simulink model "bat_cap_discharge"  (R2023a)
settings: Solver=VariableStepAuto  StartTime=0.0  StopTime=110  RelTol=1e-3
undefined symbols (not defined in the file or in its folder): Battery, Capacitor, Ri
libraries: fl_lib x41, nesl_utility x22, batteryecm_lib x1
settings Model: Creator=antaeug  LastModifiedBy=antaeug

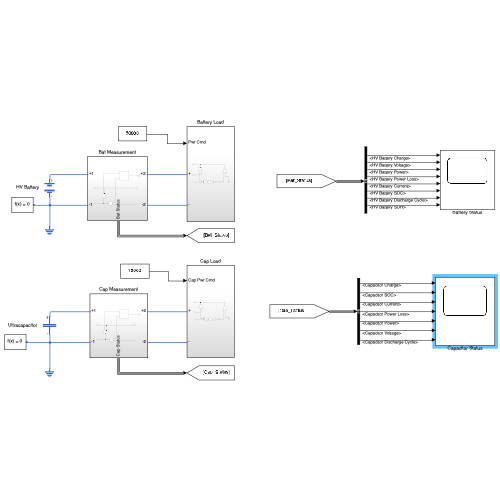
[thumbnail: Simulink's stored preview of the top-level diagram]
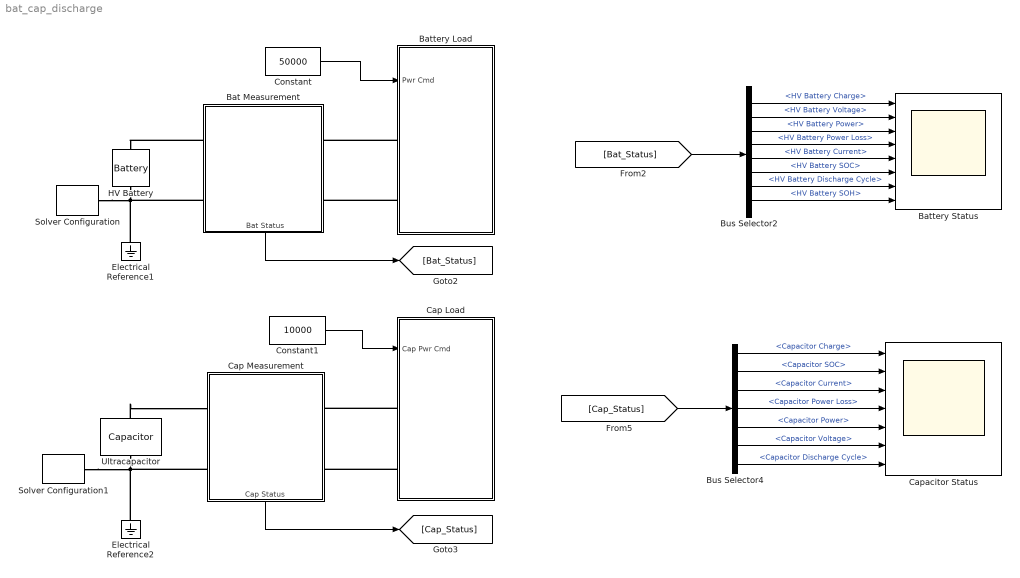
== system bat_cap_discharge ==
  Bat Measurement : Subsystem
      settings: PortSchema="{\"entries\":[{\"content\":{\"sides\":[{\"content\":{\"connectorIds\":[\"LConn1\",\"LConn2\"]},\"type\":\"ConnectorPlacement.EquallySpacedRectSide\",\"uuid\":\"d922d1f1-019d-451f-8be4-16b01e818775\"},{\"content\":{\"connectorIds\":[\"RConn1\",\"RConn2\"],\"side\":\"RIGHT\"},\"type\":\"ConnectorPlacement.EquallySpacedRectSide\",\"uuid\":\"6462d40f-4676-4bff-8e25-5b847feb4e24\"},{\"content\":{\"side\":\"TOP\"},\"type\":\"ConnectorPlacement.EquallySpacedRectSide\",\"uuid\":\"03ad4d94-013a-4b50-b094-3d1359848380\"},{\"content\":{\"connectorIds\":[\"Out1\"],\"side\":\"BOTTOM\"},\"type\":\"ConnectorPlacement.EquallySpacedRectSide\",\"uuid\":\"1e4082bc-bf86-4ee6-a4f5-78f09401198d\"}]},\"type\":\"ConnectorPlacement.EquallySpacedConnector\",\"uuid\":\"2964760f-0df3-43f8-9aa6-d9b794f3ad37\"}],\"packageUris\":[\"http://schema.mathworks.com/mf0/Connector/R2020b\"],\"version\":\"1.0\"}"
  Battery Load : Subsystem
  Battery Status : Scope  NumInputPorts=8
  Bus Selector2 : BusSelector  OutputSignals=HV Battery Charge,HV Battery Voltage,HV Battery Power,HV Battery Power Loss,HV Battery Current,HV Battery SOC,HV Battery Discharge Cycle,HV Battery SOH
  Bus Selector4 : BusSelector  OutputSignals=Capacitor Charge,Capacitor SOC,Capacitor Current,Capacitor Power Loss,Capacitor Power,Capacitor Voltage,Capacitor Discharge Cycle
  Cap Load : Subsystem
  Cap Measurement : Subsystem
      settings: PortSchema="{\"entries\":[{\"content\":{\"sides\":[{\"content\":{\"connectorIds\":[\"LConn1\",\"LConn2\"]},\"type\":\"ConnectorPlacement.EquallySpacedRectSide\",\"uuid\":\"d922d1f1-019d-451f-8be4-16b01e818775\"},{\"content\":{\"connectorIds\":[\"RConn1\",\"RConn2\"],\"side\":\"RIGHT\"},\"type\":\"ConnectorPlacement.EquallySpacedRectSide\",\"uuid\":\"6462d40f-4676-4bff-8e25-5b847feb4e24\"},{\"content\":{\"side\":\"TOP\"},\"type\":\"ConnectorPlacement.EquallySpacedRectSide\",\"uuid\":\"03ad4d94-013a-4b50-b094-3d1359848380\"},{\"content\":{\"connectorIds\":[\"Out1\"],\"side\":\"BOTTOM\"},\"type\":\"ConnectorPlacement.EquallySpacedRectSide\",\"uuid\":\"1e4082bc-bf86-4ee6-a4f5-78f09401198d\"}]},\"type\":\"ConnectorPlacement.EquallySpacedConnector\",\"uuid\":\"2964760f-0df3-43f8-9aa6-d9b794f3ad37\"}],\"packageUris\":[\"http://schema.mathworks.com/mf0/Connector/R2020b\"],\"version\":\"1.0\"}"
  Capacitor Status : Scope  NumInputPorts=7
  Constant : Constant  Value=50000
  Constant1 : Constant  Value=10000
  Electrical Reference1 : fl_lib/Electrical/Electrical Elements/Electrical Reference
  Electrical Reference2 : fl_lib/Electrical/Electrical Elements/Electrical Reference
  HV Battery : batteryecm_lib/Battery  Vnom=Battery.NominalVoltage V  prm_dir=1  R1_dis=2 Ohm  R1_ch=2 Ohm  R1=Battery.InternalResistance Ohm  prm_AH=2  AH=Battery.Capacity hr*A  V1=Battery.V1 V  AH1=Battery.AH1 hr*A  prm_R2=simscape.enum.battery.prm_R2.disabled  R2=2000 Ohm  Tmeas=25 degC  charge_measurement_port=simscape.enum.battery.enable.no  prm_dyn=simscape.enum.battery.prm_dyn.off  Rp1=0.005 Ohm  tau1=30 s  Rp2=0.005 Ohm  tau2=30 s  Rp3=0.005 Ohm  tau3=30 s  Rp4=0.005 Ohm  tau4=30 s  Rp5=0.005 Ohm  tau5=30 s  prm_fade=simscape.enum.battery.prm_fade.disabled  N_fade=100  AH_fade=45 hr*A  R1_fade=2.02 Ohm  R1_ch_fade=2.02 Ohm  V1_fade=10.35 V  prm_age=simscape.enum.battery.prm_age.disabled  prm_age_OCV=1  OCV_age=0.9  SOC_age=60  Tmeas_age=298.15 K  delta_time_age_vec=[0] d  temperature_age_vec=[273] K  OCV_scaling_age=2.2134e6  OCV_offset_age=1.632e6  temp_exp_age=0.515833569 V  t_exp_age=0.75  Vnom_T2=Vnom V  R1_T2=Ri+0.1*Ri Ohm  R1_T2_dis=2.2 Ohm  R1_T2_ch=2.2 Ohm  V1_T2=V1 V  R2_T2=2200 Ohm  Rp1_T2=0.005 Ohm  tau1_T2=30 s  Rp2_T2=0.005 Ohm  tau2_T2=30 s  Rp3_T2=0.005 Ohm  tau3_T2=30 s  Rp4_T2=0.005 Ohm  tau4_T2=30 s  Rp5_T2=0.005 Ohm  tau5_T2=30 s  Tmeas2=0 degC  thermal_port=simscape.enum.thermaleffects.omit  thermal_mass=89400 J/K  i_specify=off  i_priority=None  i=0 A  i_nominal_specify=off  i_nominal_unit=A  i_nominal_value=1  v_specify=off  v_priority=None  v=0 V  v_nominal_specify=off  v_nominal_unit=V  v_nominal_value=1  charge_specify=on  charge_priority=High  charge=Battery.InitialCharge hr*A  charge_nominal_specify=off  charge_nominal_unit=A*hr  charge_nominal_value=1  num_cycles_specify=off  num_cycles_priority=High  num_cycles=0  num_cycles_nominal_specify=off  num_cycles_nominal_unit=1  num_cycles_nominal_value=1  temperature_specify=on  temperature_priority=High  temperature=25 degC  temperature_nominal_specify=off  temperature_nominal_unit=K  temperature_nominal_value=1
  Solver Configuration : nesl_utility/Solver Configuration  PhysicalDomain=network_engine_domain  SubClassName=solver  LeftPortType=input  RightPortType=generic  Tones=[]  Harmonics=[]  SimulateNoise=off  Profile=off  UseLocalSampling=off  EnableSwitchedLinearOptims=on  FrequencyDomain=off  UseCCode=off  RelTol=0.001  AbsTol=1e-06  MinStep=1e-09  ToWorkspace=off  RevertToSquareIcSolve=off  NumHomotopyIterations=100  PhasorMode=off  PhasorModeNumHarmonics=1  ConsistencySolver=NEWTON_FTOL  IndexReductionMethod=DerivativeReplacement  DoDC=off  ResidualTolerance=1e-09  ConsistencyTolSource=GLOBAL  ConsistencyAbsTol=0.001  ConsistencyRelTol=0.001  ConsistencyTolFactor=0.001  UseLocalSolver=on  LocalSolverChoice=NE_BACKWARD_EULER_ADVANCER  ResolveIndetEquations=on  FunctionEvalNumThread=1  LocalSolverSampleTime=0.01  DoFixedCost=on  MaxNonlinIter=3  MaxModeIter=2  ComputeImpulses=off  ImpulseIterations=2  LinearAlgebra=auto  LinearAlgebraNumThread=0  EquationFormulation=NE_TIME_EF  DelaysMemoryBudget=1024  AutomaticFiltering=on  FilteringTimeConstant=0.001  PartitionStorageMethod=AS_NEEDED  PartitionMemoryBudget=1024  PartitionMethod=FAST
  Solver Configuration1 : nesl_utility/Solver Configuration  PhysicalDomain=network_engine_domain  SubClassName=solver  LeftPortType=input  RightPortType=generic  Tones=[]  Harmonics=[]  SimulateNoise=off  Profile=off  UseLocalSampling=off  EnableSwitchedLinearOptims=on  FrequencyDomain=off  UseCCode=off  RelTol=0.001  AbsTol=1e-06  MinStep=1e-09  ToWorkspace=off  RevertToSquareIcSolve=off  NumHomotopyIterations=100  PhasorMode=off  PhasorModeNumHarmonics=1  ConsistencySolver=NEWTON_FTOL  IndexReductionMethod=DerivativeReplacement  DoDC=off  ResidualTolerance=1e-09  ConsistencyTolSource=GLOBAL  ConsistencyAbsTol=0.001  ConsistencyRelTol=0.001  ConsistencyTolFactor=0.001  UseLocalSolver=on  LocalSolverChoice=NE_BACKWARD_EULER_ADVANCER  ResolveIndetEquations=on  FunctionEvalNumThread=1  LocalSolverSampleTime=0.01  DoFixedCost=on  MaxNonlinIter=3  MaxModeIter=2  ComputeImpulses=off  ImpulseIterations=2  LinearAlgebra=auto  LinearAlgebraNumThread=0  EquationFormulation=NE_TIME_EF  DelaysMemoryBudget=1024  AutomaticFiltering=on  FilteringTimeConstant=0.001  PartitionStorageMethod=AS_NEEDED  PartitionMemoryBudget=1024  PartitionMethod=FAST
  Ultracapacitor : fl_lib/Electrical/Electrical Elements/Capacitor  c=Capacitor.Capacitance F  r=Capacitor.InternalResistance mOhm  g=0 1/Ohm  i_specify=off  i_priority=None  i=20 A  i_nominal_specify=off  i_nominal_unit=A  i_nominal_value=1  v_specify=off  v_priority=None  v=600 V  v_nominal_specify=off  v_nominal_unit=V  v_nominal_value=1  vc_specify=on  vc_priority=None  vc=Capacitor.Voltage V  vc_nominal_specify=off  vc_nominal_unit=V  vc_nominal_value=600
  wires:
  Bat Measurement/1(Bat Status) -> [Bat_Status]
  Cap Measurement/1(Cap Status) -> [Cap_Status]
  Constant/1 -> Battery Load/1(Pwr Cmd)
  Constant1/1 -> Cap Load/1(Cap Pwr Cmd)
  [Bat_Status] -> Bus Selector2/1
  Bus Selector4/4 -> Capacitor Status/4  "<Capacitor Power Loss>"
  Bus Selector2/5 -> Battery Status/5  "<HV Battery Current>"
  Bus Selector2/3 -> Battery Status/3  "<HV Battery Power>"
  Bus Selector4/1 -> Capacitor Status/1  "<Capacitor Charge>"
  Bus Selector4/6 -> Capacitor Status/6  "<Capacitor Voltage>"
  Bus Selector4/2 -> Capacitor Status/2  "<Capacitor SOC>"
  Bus Selector4/3 -> Capacitor Status/3  "<Capacitor Current>"
  Bus Selector2/2 -> Battery Status/2  "<HV Battery Voltage>"
  Bus Selector2/6 -> Battery Status/6  "<HV Battery SOC>"
  Bus Selector4/5 -> Capacitor Status/5  "<Capacitor Power>"
  Bus Selector2/1 -> Battery Status/1  "<HV Battery Charge>"
  Bus Selector2/7 -> Battery Status/7  "<HV Battery Discharge Cycle>"
  Bus Selector2/4 -> Battery Status/4  "<HV Battery Power Loss>"
  Bus Selector2/8 -> Battery Status/8  "<HV Battery SOH>"
  [Cap_Status] -> Bus Selector4/1
  Bus Selector4/7 -> Capacitor Status/7  "<Capacitor Discharge Cycle>"
  connections:
  Bat Measurement/LConn2 -- HV Battery/RConn1 -- Solver Configuration/RConn1 -- Electrical Reference1/LConn1
  Cap Measurement/LConn2 -- Electrical Reference2/LConn1 -- Ultracapacitor/RConn1 -- Solver Configuration1/RConn1
  Battery Load/LConn2 -- Bat Measurement/RConn2
  Cap Load/LConn1 -- Cap Measurement/RConn1
  Battery Load/LConn1 -- Bat Measurement/RConn1
  Bat Measurement/LConn1 -- HV Battery/LConn1
  Cap Load/LConn2 -- Cap Measurement/RConn2
  Ultracapacitor/LConn1 -- Cap Measurement/LConn1

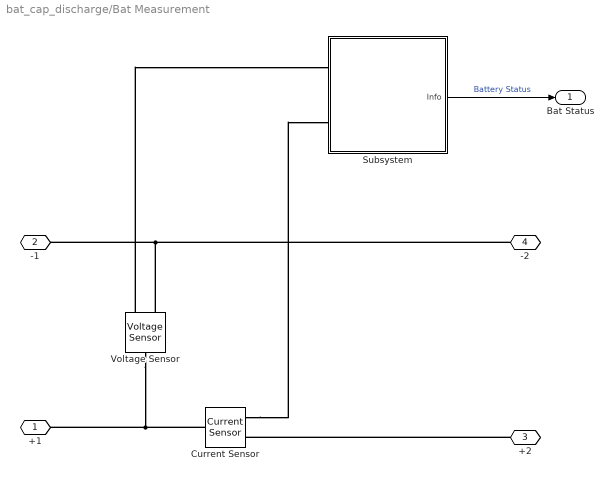
== system bat_cap_discharge/Bat Measurement ==
  Current Sensor : fl_lib/Electrical/Electrical Sensors/Current Sensor
  Subsystem : Subsystem
  Voltage Sensor : fl_lib/Electrical/Electrical Sensors/Voltage Sensor
  +1 : PMIOPort  Side=Left
  -1 : PMIOPort  Port=2  Side=Left
  +2 : PMIOPort  Port=3  Side=Right
  -2 : PMIOPort  Port=4  Side=Right
  Bat Status : Outport
  wires:
  Subsystem/1(Info) -> Bat Status/1  "Battery Status"
  connections:
  Voltage Sensor/RConn2 -- -1/RConn1 -- -2/RConn1
  Current Sensor/LConn1 -- Voltage Sensor/LConn1 -- +1/RConn1
  Voltage Sensor/RConn1 -- Subsystem/LConn1
  Current Sensor/RConn1 -- Subsystem/LConn2
  +2/RConn1 -- Current Sensor/RConn2

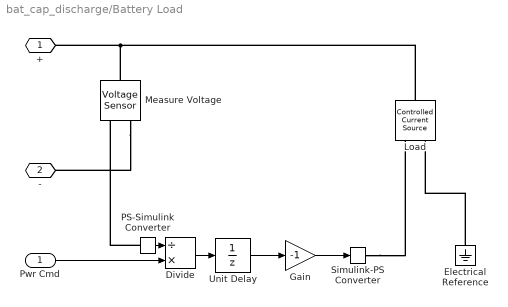
== system bat_cap_discharge/Battery Load ==
  Pwr Cmd : Inport
  Divide : Product  Inputs=/*
  Electrical Reference : fl_lib/Electrical/Electrical Elements/Electrical Reference
  Gain : Gain  Gain=-1
  Load : fl_lib/Electrical/Electrical Sources/Controlled Current Source
  Measure Voltage : fl_lib/Electrical/Electrical Sensors/Voltage Sensor
  PS-Simulink Converter : nesl_utility/PS-Simulink Converter  PhysicalDomain=network_engine_domain  SubClassName=ps_output  LeftPortType=input  RightPortType=output  PseudoPeriodic=off  Frequencies=[]  VectorFormat=inherit  Unit=V  AffineConversion=off
  Simulink-PS Converter : nesl_utility/Simulink-PS Converter  PhysicalDomain=network_engine_domain  SubClassName=ps_input  LeftPortType=input  RightPortType=output  PseudoPeriodic=off  Frequencies=[]  NoiseDistribution=none  NoiseParameters=[]  Unit=A  AffineConversion=off  FilteringAndDerivatives=provide  SimscapeFilterOrder=1  InputFilterTimeConstant=0.001  UdotUserProvided=0
  Unit Delay : UnitDelay  SampleTime=-1  HasFrameUpgradeWarning=on
  + : PMIOPort  Side=Left
  - : PMIOPort  Port=2  Side=Left
  wires:
  PS-Simulink Converter/1 -> Divide/1
  Pwr Cmd/1 -> Divide/2
  Divide/1 -> Unit Delay/1
  Unit Delay/1 -> Gain/1
  Gain/1 -> Simulink-PS Converter/1
  connections:
  Electrical Reference/LConn1 -- Load/RConn2
  Load/LConn1 -- Measure Voltage/LConn1 -- +/RConn1
  Measure Voltage/RConn2 -- -/RConn1
  PS-Simulink Converter/LConn1 -- Measure Voltage/RConn1
  Simulink-PS Converter/RConn1 -- Load/RConn1

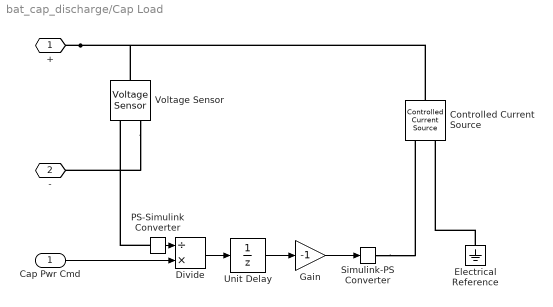
== system bat_cap_discharge/Cap Load ==
  Cap Pwr Cmd : Inport
  Controlled Current Source : fl_lib/Electrical/Electrical Sources/Controlled Current Source
  Divide : Product  Inputs=/*
  Electrical Reference : fl_lib/Electrical/Electrical Elements/Electrical Reference
  Gain : Gain  Gain=-1
  PS-Simulink Converter : nesl_utility/PS-Simulink Converter  PhysicalDomain=network_engine_domain  SubClassName=ps_output  LeftPortType=input  RightPortType=output  PseudoPeriodic=off  Frequencies=[]  VectorFormat=inherit  Unit=V  AffineConversion=off
  Simulink-PS Converter : nesl_utility/Simulink-PS Converter  PhysicalDomain=network_engine_domain  SubClassName=ps_input  LeftPortType=input  RightPortType=output  PseudoPeriodic=off  Frequencies=[]  NoiseDistribution=none  NoiseParameters=[]  Unit=A  AffineConversion=off  FilteringAndDerivatives=provide  SimscapeFilterOrder=1  InputFilterTimeConstant=0.001  UdotUserProvided=0
  Unit Delay : UnitDelay  SampleTime=-1  HasFrameUpgradeWarning=on
  Voltage Sensor : fl_lib/Electrical/Electrical Sensors/Voltage Sensor
  + : PMIOPort  Side=Left
  - : PMIOPort  Port=2  Side=Left
  wires:
  PS-Simulink Converter/1 -> Divide/1
  Cap Pwr Cmd/1 -> Divide/2
  Divide/1 -> Unit Delay/1
  Unit Delay/1 -> Gain/1
  Gain/1 -> Simulink-PS Converter/1
  connections:
  Electrical Reference/LConn1 -- Controlled Current Source/RConn2
  +/RConn1 -- Controlled Current Source/LConn1 -- Voltage Sensor/LConn1
  Voltage Sensor/RConn2 -- -/RConn1
  PS-Simulink Converter/LConn1 -- Voltage Sensor/RConn1
  Simulink-PS Converter/RConn1 -- Controlled Current Source/RConn1

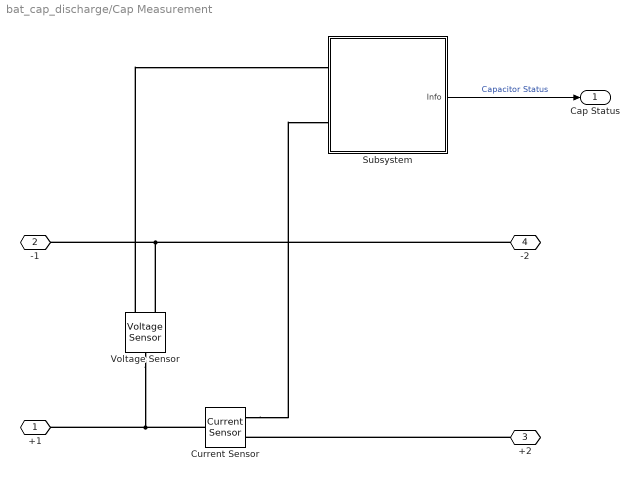
== system bat_cap_discharge/Cap Measurement ==
  Current Sensor : fl_lib/Electrical/Electrical Sensors/Current Sensor
  Subsystem : Subsystem
  Voltage Sensor : fl_lib/Electrical/Electrical Sensors/Voltage Sensor
  +1 : PMIOPort  Side=Left
  -1 : PMIOPort  Port=2  Side=Left
  +2 : PMIOPort  Port=3  Side=Right
  -2 : PMIOPort  Port=4  Side=Right
  Cap Status : Outport
  wires:
  Subsystem/1(Info) -> Cap Status/1  "Capacitor Status"
  connections:
  -2/RConn1 -- Voltage Sensor/RConn2 -- -1/RConn1
  Current Sensor/LConn1 -- Voltage Sensor/LConn1 -- +1/RConn1
  Voltage Sensor/RConn1 -- Subsystem/LConn1
  Current Sensor/RConn1 -- Subsystem/LConn2
  +2/RConn1 -- Current Sensor/RConn2

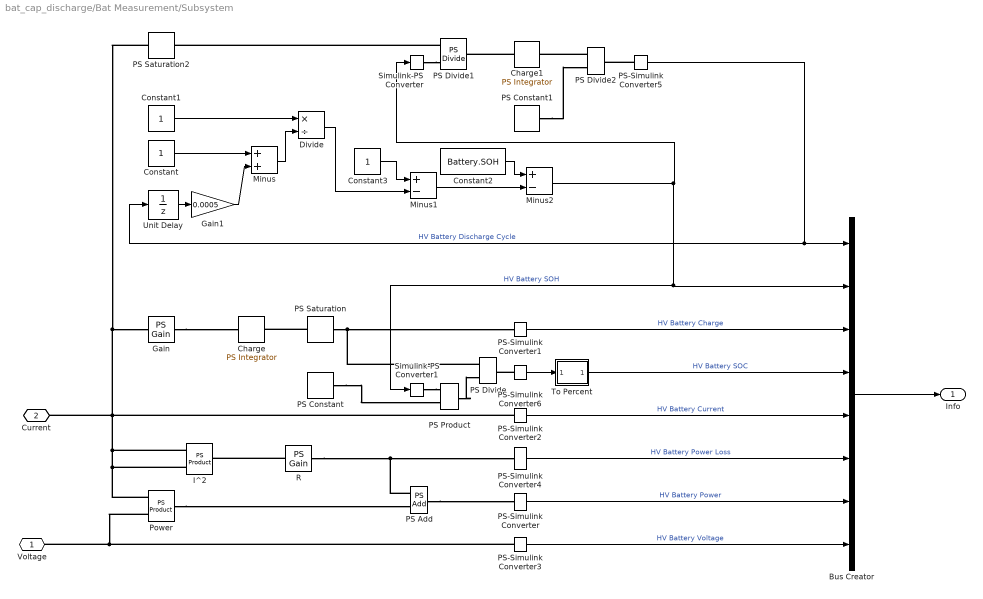
== system bat_cap_discharge/Bat Measurement/Subsystem ==
  Bus Creator : BusCreator  Inputs=8
  Charge : fl_lib/Physical Signals/Linear Operators/PS Integrator  reset_method=foundation.enum.IntegratorResetSpec.None  initial_condition_spec=foundation.enum.IntegratorICSpec.Internal  saturation_spec=foundation.enum.IntegratorSaturationSpec.None  saturation_source_spec=foundation.enum.IntegratorSaturationSourceSpec.Internal  x0=Battery.InitialCharge A*hr  xu=inf s  xl=-inf s
      settings: AttributesFormatString=%<x0> [%<x0_unit>]
  Charge1 : fl_lib/Physical Signals/Linear Operators/PS Integrator  reset_method=foundation.enum.IntegratorResetSpec.None  initial_condition_spec=foundation.enum.IntegratorICSpec.Internal  saturation_spec=foundation.enum.IntegratorSaturationSpec.None  saturation_source_spec=foundation.enum.IntegratorSaturationSourceSpec.Internal  x0=0 A*hr  xu=inf s  xl=-inf s
      settings: AttributesFormatString=%<x0> [%<x0_unit>]
  Constant : Constant
  Constant1 : Constant
  Constant2 : Constant  Value=Battery.SOH
  Constant3 : Constant
  Divide : Product  Inputs=*/
  Gain : fl_lib/Physical Signals/Functions/PS Gain  gain=-1
      settings: AttributesFormatString=%<gain>
  Gain1 : Gain  Gain=0.0005
  I^2 : fl_lib/Physical Signals/Functions/PS Product
  Minus : Sum
  Minus1 : Sum  Inputs=+-
  Minus2 : Sum  Inputs=+-
  PS Add : fl_lib/Physical Signals/Functions/PS Add
  PS Constant : fl_lib/Physical Signals/Sources/PS Constant  constant=Battery.Capacity A*hr
      settings: AttributesFormatString=%<constant> [%<constant_unit>]
  PS Constant1 : fl_lib/Physical Signals/Sources/PS Constant  constant=Battery.Capacity A*hr
  PS Divide : fl_lib/Physical Signals/Functions/PS Divide
  PS Divide1 : fl_lib/Physical Signals/Functions/PS Divide
  PS Divide2 : fl_lib/Physical Signals/Functions/PS Divide
  PS Product : fl_lib/Physical Signals/Functions/PS Product
  PS Saturation : fl_lib/Physical Signals/Nonlinear Operators/PS Saturation  upper_limit=Battery.Capacity A*hr  lower_limit=0 A*hr
      settings: AttributesFormatString=|
      | Upper: %<upper_limit>
      | Lower: %<lower_limit>
  PS Saturation2 : fl_lib/Physical Signals/Nonlinear Operators/PS Saturation  upper_limit=500 A  lower_limit=0 A
  PS-Simulink Converter : nesl_utility/PS-Simulink Converter  PhysicalDomain=network_engine_domain  SubClassName=ps_output  LeftPortType=input  RightPortType=output  PseudoPeriodic=off  Frequencies=[]  VectorFormat=1-D array  Unit=W  AffineConversion=off
  PS-Simulink Converter1 : nesl_utility/PS-Simulink Converter  PhysicalDomain=network_engine_domain  SubClassName=ps_output  LeftPortType=input  RightPortType=output  PseudoPeriodic=off  Frequencies=[]  VectorFormat=1-D array  Unit=A*hr  AffineConversion=off
  PS-Simulink Converter2 : nesl_utility/PS-Simulink Converter  PhysicalDomain=network_engine_domain  SubClassName=ps_output  LeftPortType=input  RightPortType=output  PseudoPeriodic=off  Frequencies=[]  VectorFormat=1-D array  Unit=A  AffineConversion=off
  PS-Simulink Converter3 : nesl_utility/PS-Simulink Converter  PhysicalDomain=network_engine_domain  SubClassName=ps_output  LeftPortType=input  RightPortType=output  PseudoPeriodic=off  Frequencies=[]  VectorFormat=1-D array  Unit=V  AffineConversion=off
  PS-Simulink Converter4 : nesl_utility/PS-Simulink Converter  PhysicalDomain=network_engine_domain  SubClassName=ps_output  LeftPortType=input  RightPortType=output  PseudoPeriodic=off  Frequencies=[]  VectorFormat=1-D array  Unit=W  AffineConversion=off
  PS-Simulink Converter5 : nesl_utility/PS-Simulink Converter  PhysicalDomain=network_engine_domain  SubClassName=ps_output  LeftPortType=input  RightPortType=output  PseudoPeriodic=off  Frequencies=[]  VectorFormat=inherit  Unit=1  AffineConversion=off
  PS-Simulink Converter6 : nesl_utility/PS-Simulink Converter  PhysicalDomain=network_engine_domain  SubClassName=ps_output  LeftPortType=input  RightPortType=output  PseudoPeriodic=off  Frequencies=[]  VectorFormat=1-D array  Unit=1  AffineConversion=off
  Power : fl_lib/Physical Signals/Functions/PS Product
  R : fl_lib/Physical Signals/Functions/PS Gain  gain=Battery.InternalResistance Ohm
      settings: AttributesFormatString=%<gain> [%<gain_unit>]
  Simulink-PS Converter : nesl_utility/Simulink-PS Converter  PhysicalDomain=network_engine_domain  SubClassName=ps_input  LeftPortType=input  RightPortType=output  PseudoPeriodic=off  Frequencies=[]  NoiseDistribution=none  NoiseParameters=[]  Unit=1  AffineConversion=off  FilteringAndDerivatives=provide  SimscapeFilterOrder=1  InputFilterTimeConstant=0.001  UdotUserProvided=0
  Simulink-PS Converter1 : nesl_utility/Simulink-PS Converter  PhysicalDomain=network_engine_domain  SubClassName=ps_input  LeftPortType=input  RightPortType=output  PseudoPeriodic=off  Frequencies=[]  NoiseDistribution=none  NoiseParameters=[]  Unit=1  AffineConversion=off  FilteringAndDerivatives=provide  SimscapeFilterOrder=1  InputFilterTimeConstant=0.001  UdotUserProvided=0
  To Percent : Subsystem
  Unit Delay : UnitDelay  SampleTime=-1  HasFrameUpgradeWarning=on
  Voltage : PMIOPort  Side=Left
  Current : PMIOPort  Port=2  Side=Left
  Info : Outport
  wires:
  PS-Simulink Converter4/1 -> Bus Creator/6  "HV Battery Power Loss"
  PS-Simulink Converter3/1 -> Bus Creator/8  "HV Battery Voltage"
  PS-Simulink Converter1/1 -> Bus Creator/3  "HV Battery Charge"
  Bus Creator/1 -> Info/1
  To Percent/1(Out1) -> Bus Creator/4  "HV Battery SOC"
  PS-Simulink Converter/1 -> Bus Creator/7  "HV Battery Power"
  PS-Simulink Converter6/1 -> To Percent/1(In1)
  PS-Simulink Converter2/1 -> Bus Creator/5  "HV Battery Current"
  Constant/1 -> Minus/1
  Gain1/1 -> Minus/2
  Unit Delay/1 -> Gain1/1
  Divide/1 -> Minus1/2
  Constant1/1 -> Divide/1
  Minus/1 -> Divide/2
  PS-Simulink Converter5/1 -> Bus Creator/1, Unit Delay/1  "HV Battery Discharge Cycle"
  Constant3/1 -> Minus1/1
  Constant2/1 -> Minus2/1
  Minus1/1 -> Minus2/2
  Minus2/1 -> Simulink-PS Converter1/1, Bus Creator/2, Simulink-PS Converter/1  "HV Battery SOH"
  connections:
  PS Divide/LConn1 -- PS-Simulink Converter1/LConn1 -- PS Saturation/RConn1
  Power/LConn1 -- Voltage/RConn1 -- PS-Simulink Converter3/LConn1
  R/RConn1 -- PS Add/LConn1 -- PS-Simulink Converter4/LConn1
  Power/LConn2 -- I^2/LConn1 -- Current/RConn1 -- PS Saturation2/LConn1 -- Gain/LConn1 -- PS-Simulink Converter2/LConn1 -- I^2/LConn2
  PS Add/RConn1 -- PS-Simulink Converter/LConn1
  R/LConn1 -- I^2/RConn1
  PS Saturation/LConn1 -- Charge/RConn1
  Gain/RConn1 -- Charge/LConn1
  PS-Simulink Converter6/LConn1 -- PS Divide/RConn1
  Power/RConn1 -- PS Add/LConn2
  PS Divide1/LConn1 -- PS Saturation2/RConn1
  Charge1/LConn1 -- PS Divide1/RConn1
  PS Divide2/LConn1 -- Charge1/RConn1
  PS Constant1/RConn1 -- PS Divide2/LConn2
  PS-Simulink Converter5/LConn1 -- PS Divide2/RConn1
  Simulink-PS Converter/RConn1 -- PS Divide1/LConn2
  PS Product/RConn1 -- PS Divide/LConn2
  PS Constant/RConn1 -- PS Product/LConn2
  Simulink-PS Converter1/RConn1 -- PS Product/LConn1

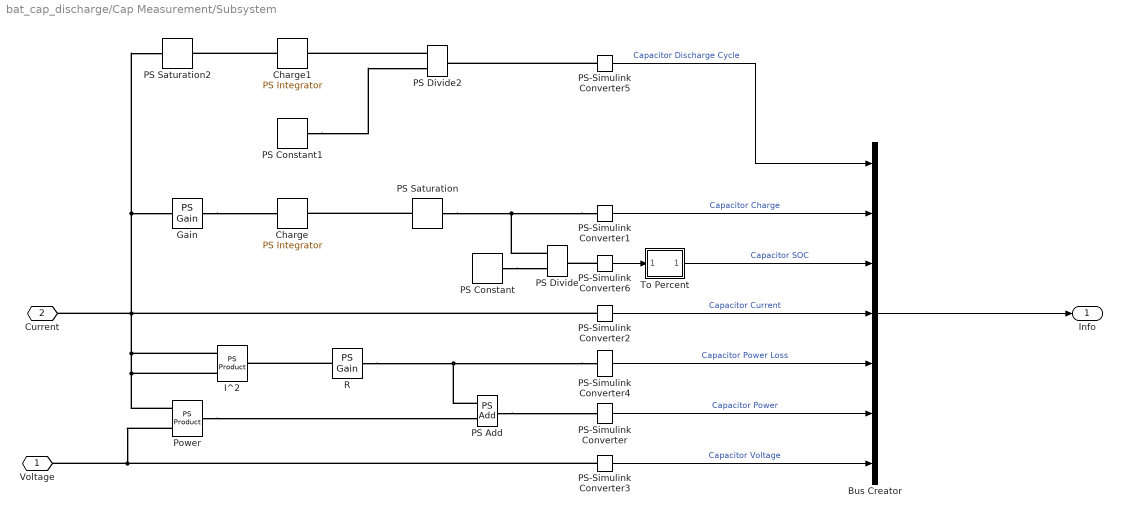
== system bat_cap_discharge/Cap Measurement/Subsystem ==
  Bus Creator : BusCreator  Inputs=7
  Charge : fl_lib/Physical Signals/Linear Operators/PS Integrator  reset_method=foundation.enum.IntegratorResetSpec.None  initial_condition_spec=foundation.enum.IntegratorICSpec.Internal  saturation_spec=foundation.enum.IntegratorSaturationSpec.None  saturation_source_spec=foundation.enum.IntegratorSaturationSourceSpec.Internal  x0=Capacitor.Capacity A*hr  xu=inf s  xl=-inf s
      settings: AttributesFormatString=%<x0> [%<x0_unit>]
  Charge1 : fl_lib/Physical Signals/Linear Operators/PS Integrator  reset_method=foundation.enum.IntegratorResetSpec.None  initial_condition_spec=foundation.enum.IntegratorICSpec.Internal  saturation_spec=foundation.enum.IntegratorSaturationSpec.None  saturation_source_spec=foundation.enum.IntegratorSaturationSourceSpec.Internal  x0=0 A*hr  xu=inf s  xl=-inf s
      settings: AttributesFormatString=%<x0> [%<x0_unit>]
  Gain : fl_lib/Physical Signals/Functions/PS Gain  gain=-1
      settings: AttributesFormatString=%<gain>
  I^2 : fl_lib/Physical Signals/Functions/PS Product
  PS Add : fl_lib/Physical Signals/Functions/PS Add
  PS Constant : fl_lib/Physical Signals/Sources/PS Constant  constant=Capacitor.Capacity A*hr
      settings: AttributesFormatString=%<constant> [%<constant_unit>]
  PS Constant1 : fl_lib/Physical Signals/Sources/PS Constant  constant=Capacitor.Capacity A*hr
      settings: AttributesFormatString=%<constant> [%<constant_unit>]
  PS Divide : fl_lib/Physical Signals/Functions/PS Divide
  PS Divide2 : fl_lib/Physical Signals/Functions/PS Divide
  PS Saturation : fl_lib/Physical Signals/Nonlinear Operators/PS Saturation  upper_limit=Capacitor.Capacity A*hr  lower_limit=0 A*hr
      settings: AttributesFormatString=|
      | Upper: %<upper_limit>
      | Lower: %<lower_limit>
  PS Saturation2 : fl_lib/Physical Signals/Nonlinear Operators/PS Saturation  upper_limit=500 A  lower_limit=0 A
  PS-Simulink Converter : nesl_utility/PS-Simulink Converter  PhysicalDomain=network_engine_domain  SubClassName=ps_output  LeftPortType=input  RightPortType=output  PseudoPeriodic=off  Frequencies=[]  VectorFormat=1-D array  Unit=W  AffineConversion=off
  PS-Simulink Converter1 : nesl_utility/PS-Simulink Converter  PhysicalDomain=network_engine_domain  SubClassName=ps_output  LeftPortType=input  RightPortType=output  PseudoPeriodic=off  Frequencies=[]  VectorFormat=1-D array  Unit=A*hr  AffineConversion=off
  PS-Simulink Converter2 : nesl_utility/PS-Simulink Converter  PhysicalDomain=network_engine_domain  SubClassName=ps_output  LeftPortType=input  RightPortType=output  PseudoPeriodic=off  Frequencies=[]  VectorFormat=1-D array  Unit=A  AffineConversion=off
  PS-Simulink Converter3 : nesl_utility/PS-Simulink Converter  PhysicalDomain=network_engine_domain  SubClassName=ps_output  LeftPortType=input  RightPortType=output  PseudoPeriodic=off  Frequencies=[]  VectorFormat=1-D array  Unit=V  AffineConversion=off
  PS-Simulink Converter4 : nesl_utility/PS-Simulink Converter  PhysicalDomain=network_engine_domain  SubClassName=ps_output  LeftPortType=input  RightPortType=output  PseudoPeriodic=off  Frequencies=[]  VectorFormat=1-D array  Unit=W  AffineConversion=off
  PS-Simulink Converter5 : nesl_utility/PS-Simulink Converter  PhysicalDomain=network_engine_domain  SubClassName=ps_output  LeftPortType=input  RightPortType=output  PseudoPeriodic=off  Frequencies=[]  VectorFormat=inherit  Unit=1  AffineConversion=off
  PS-Simulink Converter6 : nesl_utility/PS-Simulink Converter  PhysicalDomain=network_engine_domain  SubClassName=ps_output  LeftPortType=input  RightPortType=output  PseudoPeriodic=off  Frequencies=[]  VectorFormat=1-D array  Unit=1  AffineConversion=off
  Power : fl_lib/Physical Signals/Functions/PS Product
  R : fl_lib/Physical Signals/Functions/PS Gain  gain=Capacitor.InternalResistance Ohm
      settings: AttributesFormatString=%<gain> [%<gain_unit>]
  To Percent : Subsystem
  Voltage : PMIOPort  Side=Left
  Current : PMIOPort  Port=2  Side=Left
  Info : Outport
  wires:
  PS-Simulink Converter4/1 -> Bus Creator/5  "Capacitor Power Loss"
  PS-Simulink Converter3/1 -> Bus Creator/7  "Capacitor Voltage"
  PS-Simulink Converter1/1 -> Bus Creator/2  "Capacitor Charge"
  Bus Creator/1 -> Info/1
  To Percent/1(Out1) -> Bus Creator/3  "Capacitor SOC"
  PS-Simulink Converter/1 -> Bus Creator/6  "Capacitor Power"
  PS-Simulink Converter6/1 -> To Percent/1(In1)
  PS-Simulink Converter2/1 -> Bus Creator/4  "Capacitor Current"
  PS-Simulink Converter5/1 -> Bus Creator/1  "Capacitor Discharge Cycle"
  connections:
  PS-Simulink Converter1/LConn1 -- PS Divide/LConn1 -- PS Saturation/RConn1
  PS-Simulink Converter3/LConn1 -- Power/LConn1 -- Voltage/RConn1
  PS-Simulink Converter4/LConn1 -- R/RConn1 -- PS Add/LConn1
  Current/RConn1 -- PS Saturation2/LConn1 -- Gain/LConn1 -- PS-Simulink Converter2/LConn1 -- I^2/LConn2 -- I^2/LConn1 -- Power/LConn2
  PS Add/RConn1 -- PS-Simulink Converter/LConn1
  R/LConn1 -- I^2/RConn1
  PS Saturation/LConn1 -- Charge/RConn1
  Gain/RConn1 -- Charge/LConn1
  PS-Simulink Converter6/LConn1 -- PS Divide/RConn1
  Power/RConn1 -- PS Add/LConn2
  PS Constant/RConn1 -- PS Divide/LConn2
  Charge1/LConn1 -- PS Saturation2/RConn1
  PS-Simulink Converter5/LConn1 -- PS Divide2/RConn1
  PS Divide2/LConn1 -- Charge1/RConn1
  PS Constant1/RConn1 -- PS Divide2/LConn2

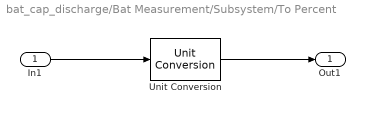
== system bat_cap_discharge/Bat Measurement/Subsystem/To Percent ==
  In1 : Inport
  Unit Conversion : UnitConversion
  Out1 : Outport  Unit=%
      settings: AttributesFormatString=%<Unit>
  wires:
  Unit Conversion/1 -> Out1/1
  In1/1 -> Unit Conversion/1

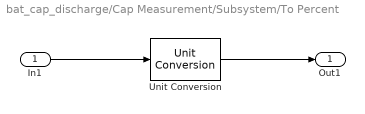
== system bat_cap_discharge/Cap Measurement/Subsystem/To Percent ==
  In1 : Inport
  Unit Conversion : UnitConversion
  Out1 : Outport  Unit=%
      settings: AttributesFormatString=%<Unit>
  wires:
  Unit Conversion/1 -> Out1/1
  In1/1 -> Unit Conversion/1
